simulink model "serializer"  (R2019b)
settings: Solver=VariableStepAuto  StartTime=0.0  StopTime=30  RelTol=1e-3
InitFcn:
  | %% DSPBuilder Start
  | alt_dspbuilder_update_model(bdroot)
  | %% DSPBuilder End
  | 
  | serializer_init
StartFcn:
  | %% DSPBuilder Start
  | alt_dspbuilder_hdlimport_prepare_for_simulation(bdroot)
  | %% DSPBuilder End
StopFcn:
  | serializer_analysis
libraries: allblocks_alteradspbuilder2 x15, dspsrcs4 x2
settings Model: Creator=vboxuser  LastModifiedBy=vboxuser

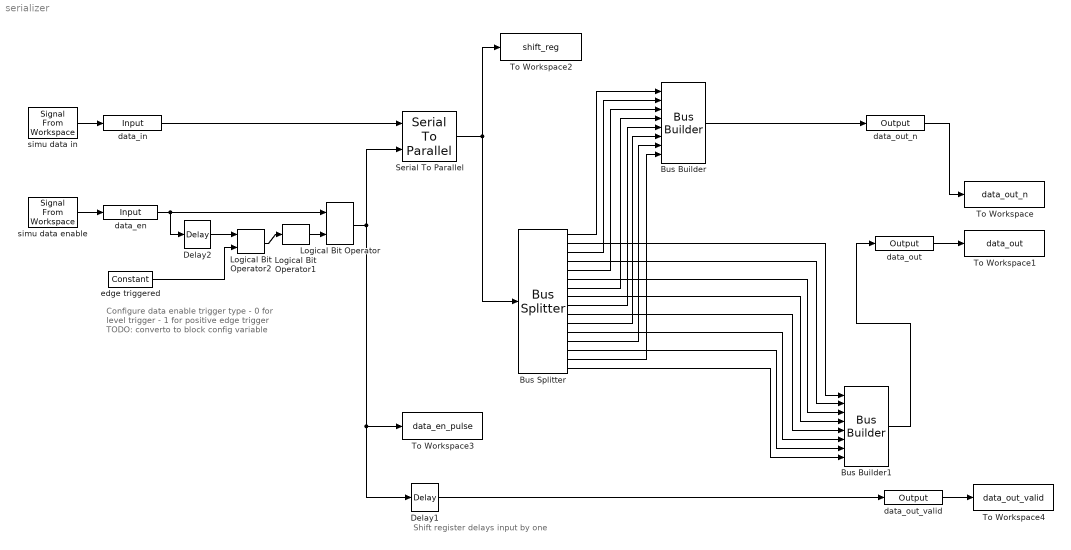
== system serializer ==
  note: Shift register delays input by one
  note: Configure data enable trigger type
      |  - 0 for level trigger
      |  - 1 for positive edge trigger
      |
      | TODO: converto to block config variable
  Bus Builder : allblocks_alteradspbuilder2/Bus Builder  BusType=Signed Integer  bwl=8  bwr=1  pipeline_display=0
  Bus Builder1 : allblocks_alteradspbuilder2/Bus Builder  BusType=Signed Integer  bwl=8  bwr=1  pipeline_display=0
  Bus Splitter : allblocks_alteradspbuilder2/Bus Splitter  BusType=Unsigned Integer  bwl=16  bwr=0  pipeline_display=0
  Delay1 : allblocks_alteradspbuilder2/Delay  pipeline=1  pipeline_display=1  ClockPhase=1  use_ena=off  use_sclr=off  allowFloatingPointOverride=on  logOutputs=off  logFile=C:\Users\vboxuser\Documents\MATLAB\serializer\tb_serializer\serializer_Delay1.fixedpointlog  use_init=off  reset_value=1
  Delay2 : allblocks_alteradspbuilder2/Delay  pipeline=1  pipeline_display=1  ClockPhase=1  use_ena=off  use_sclr=off  allowFloatingPointOverride=on  logOutputs=off  logFile=C:\Users\vboxuser\Documents\MATLAB\serializer\tb_serializer\serializer_Delay2.fixedpointlog  use_init=off  reset_value=1
  Logical Bit Operator : allblocks_alteradspbuilder2/Logical Bit Operator  LogicalOperator=AND  user_inputs=2  pipeline_display=0
  Logical Bit Operator1 : allblocks_alteradspbuilder2/Logical Bit Operator  LogicalOperator=NOT  user_inputs=2  pipeline_display=0
  Logical Bit Operator2 : allblocks_alteradspbuilder2/Logical Bit Operator  LogicalOperator=AND  user_inputs=2  pipeline_display=0
  Serial To Parallel : allblocks_alteradspbuilder2/Serial To Parallel  BusType=Unsigned Integer  bwl=16  bwr=0  msbfirsttext=MSB First  msbfirst=1  use_ena=on  use_sclr=off
  To Workspace : ToWorkspace  VariableName=data_out_n  SampleTime=-1
      settings: Save2DSignal=2-D array (concatenate along first dimension)
  To Workspace1 : ToWorkspace  VariableName=data_out  SampleTime=-1
      settings: Save2DSignal=2-D array (concatenate along first dimension)
  To Workspace2 : ToWorkspace  VariableName=shift_reg  SampleTime=-1
      settings: Save2DSignal=2-D array (concatenate along first dimension)
  To Workspace3 : ToWorkspace  VariableName=data_en_pulse  SampleTime=-1
      settings: Save2DSignal=2-D array (concatenate along first dimension)
  To Workspace4 : ToWorkspace  VariableName=data_out_valid  SampleTime=-1
      settings: Save2DSignal=2-D array (concatenate along first dimension)
  data_en : allblocks_alteradspbuilder2/Input  iofile=C:\Users\vboxuser\Documents\MATLAB\serializer\tb_serializer\serializer_data%5Fen.salt  BusType=Single Bit  bwl=8  bwr=0  SpecifyClock=off  PORTTYPE=Input  externalType=Inferred  allowFloatingPointOverride=on  logOutputs=off
  data_in : allblocks_alteradspbuilder2/Input  iofile=C:\Users\vboxuser\Documents\MATLAB\serializer\tb_serializer\serializer_data%5Fin.salt  BusType=Single Bit  bwl=1  bwr=0  SpecifyClock=off  PORTTYPE=Input  externalType=Inferred  allowFloatingPointOverride=on  logOutputs=off
  data_out : allblocks_alteradspbuilder2/Output  iofile=C:\Users\vboxuser\Documents\MATLAB\serializer\tb_serializer\serializer_data%5Fout.capture  BusType=Unsigned Integer  bwl=8  bwr=0  externalType=Inferred  PORTTYPE=Output  allowFloatingPointOverride=on  logOutputs=off
  data_out_n : allblocks_alteradspbuilder2/Output  iofile=C:\Users\vboxuser\Documents\MATLAB\serializer\tb_serializer\serializer_data%5Fout%5Fn.capture  BusType=Unsigned Integer  bwl=8  bwr=0  externalType=Inferred  PORTTYPE=Output  allowFloatingPointOverride=on  logOutputs=off
  data_out_valid : allblocks_alteradspbuilder2/Output  iofile=C:\Users\vboxuser\Documents\MATLAB\serializer\tb_serializer\serializer_data%5Fout%5Fvalid.capture  BusType=Single Bit  bwl=8  bwr=0  externalType=Inferred  PORTTYPE=Output  allowFloatingPointOverride=on  logOutputs=off
  edge triggered : allblocks_alteradspbuilder2/Constant  mask_cst=0  BusType=Single Bit  bwl=8  bwr=0  roundMode=Truncate  satMode=Wrap  SpecifyClock=off  allowFloatingPointOverride=on  logOutputs=off  logFile=C:\Users\vboxuser\Documents\MATLAB\serializer\tb_serializer\serializer_edge+triggered.fixedpointlog
  simu data enable : dspsrcs4/Signal From Workspace  X=data_en  Ts=1  nsamps=1  OutputAfterFinalValue=Setting to zero  ignoreOrWarnInputAndFrameLengths=off  OutputFrames=off
  simu data in : dspsrcs4/Signal From Workspace  X=data_in  Ts=1  nsamps=1  OutputAfterFinalValue=Setting to zero  ignoreOrWarnInputAndFrameLengths=off  OutputFrames=off
  wires:
  data_in/1 -> Serial To Parallel/1
  data_en/1 -> Logical Bit Operator/1, Delay2/1
  Serial To Parallel/1 -> Bus Splitter/1, To Workspace2/1
  Delay2/1 -> Logical Bit Operator2/1
  Logical Bit Operator/1 -> To Workspace3/1, Delay1/1, Serial To Parallel/2
  simu data in/1 -> data_in/1
  simu data enable/1 -> data_en/1
  data_out_n/1 -> To Workspace/1
  data_out/1 -> To Workspace1/1
  edge triggered/1 -> Logical Bit Operator2/2
  Logical Bit Operator1/1 -> Logical Bit Operator/2
  Logical Bit Operator2/1 -> Logical Bit Operator1/1
  Delay1/1 -> data_out_valid/1
  data_out_valid/1 -> To Workspace4/1
  Bus Splitter/1 -> Bus Builder/1
  Bus Splitter/3 -> Bus Builder/2
  Bus Splitter/5 -> Bus Builder/3
  Bus Splitter/7 -> Bus Builder/4
  Bus Splitter/9 -> Bus Builder/5
  Bus Splitter/10 -> Bus Builder1/5
  Bus Splitter/11 -> Bus Builder/6
  Bus Splitter/13 -> Bus Builder/7
  Bus Splitter/15 -> Bus Builder/8
  Bus Splitter/2 -> Bus Builder1/1
  Bus Splitter/4 -> Bus Builder1/2
  Bus Splitter/6 -> Bus Builder1/3
  Bus Splitter/8 -> Bus Builder1/4
  Bus Splitter/12 -> Bus Builder1/6
  Bus Splitter/14 -> Bus Builder1/7
  Bus Splitter/16 -> Bus Builder1/8
  Bus Builder/1 -> data_out_n/1
  Bus Builder1/1 -> data_out/1
